simulink model "Prp_TrqDesCoord1"  (R2016b)
settings: configuration reference "CodeGenConfigSet" (kept outside this file)
settings Model: Creator=Wollf  LastModifiedBy=Wollf
settings ConfigSetRef: SourceLocation=Base Workspace

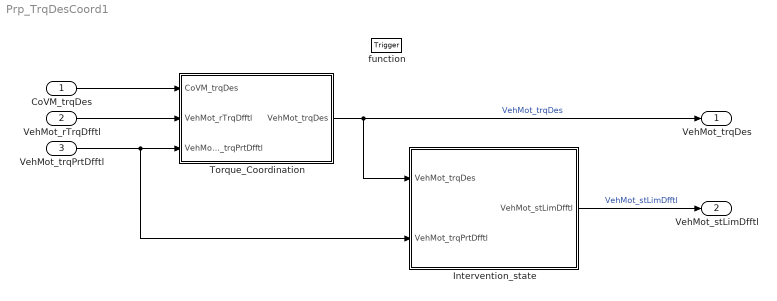
== system Prp_TrqDesCoord1 ==
  CoVM_trqDes : Inport  Tag=Nm  Description=Propulsion torque order after ESP-torque intervention coordination (wheel torque)  OutMin=-3000  OutMax=3000  OutDataTypeStr=Trq_Nm
  VehMot_rTrqDfftl : Inport  Description=Torque ratio of differential  Port=2  OutMin=-300  OutMax=300  OutDataTypeStr=TransRatio
  VehMot_trqPrtDfftl : Inport  Tag=Nm  Description=Differential protection torque  Port=3  OutMin=-3000  OutMax=3000  OutDataTypeStr=Trq_Nm
  function : TriggerPort  TriggerType=function-call  VariantControl=Variant
  Intervention_state : Subsystem
  Torque_Coordination : Subsystem
  VehMot_trqDes : Outport  Tag=Nm  Description=Desired torque for propulsion (transmission output torque)  OutMin=-3000  OutMax=3000  OutDataTypeStr=Trq_Nm
  VehMot_stLimDfftl : Outport  Description=Status torque intervention differential protection  Port=2  OutMin=0  OutMax=255  OutDataTypeStr=State_uint8
  wires:
  Intervention_state/1(VehMot_stLimDfftl) -> VehMot_stLimDfftl/1  "VehMot_stLimDfftl"
  CoVM_trqDes/1 -> Torque_Coordination/1(CoVM_trqDes)
  VehMot_rTrqDfftl/1 -> Torque_Coordination/2(VehMot_rTrqDfftl)
  VehMot_trqPrtDfftl/1 -> Intervention_state/2(VehMot_trqPrtDfftl), Torque_Coordination/3(VehMot_trqPrtDfftl)
  Torque_Coordination/1(VehMot_trqDes) -> VehMot_trqDes/1, Intervention_state/1(VehMot_trqDes)  "VehMot_trqDes"

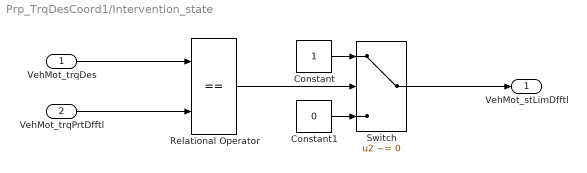
== system Prp_TrqDesCoord1/Intervention_state ==
  VehMot_trqDes : Inport
  VehMot_trqPrtDfftl : Inport  Port=2
  Constant : Constant  OutDataTypeStr=Inherit: Inherit via back propagation
  Constant1 : Constant  Value=0  OutDataTypeStr=Inherit: Inherit via back propagation
  Relational Operator : RelationalOperator  Operator===  OutDataTypeStr=boolean  RndMeth=Simplest  InputSameDT=on
  Switch : Switch  Criteria=u2 ~= 0  InputSameDT=on
  VehMot_stLimDfftl : Outport
  wires:
  Switch/1 -> VehMot_stLimDfftl/1
  Constant1/1 -> Switch/3
  Constant/1 -> Switch/1
  Relational Operator/1 -> Switch/2
  VehMot_trqPrtDfftl/1 -> Relational Operator/2
  VehMot_trqDes/1 -> Relational Operator/1

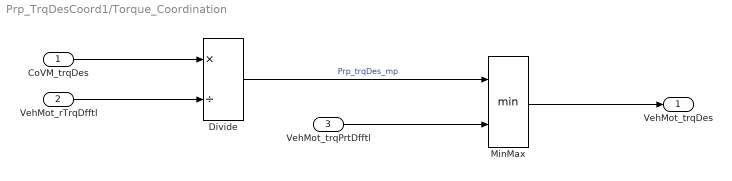
== system Prp_TrqDesCoord1/Torque_Coordination ==
  CoVM_trqDes : Inport  Tag=Nm  Description=Propulsion torque order after ESP-torque intervention coordination (wheel torque)  OutMin=-3000  OutMax=3000  OutDataTypeStr=Trq_Nm
  VehMot_rTrqDfftl : Inport  Tag=-  Description=Torque ratio of differential  Port=2  OutMin=-300  OutMax=300  OutDataTypeStr=TransRatio
  VehMot_trqPrtDfftl : Inport  Tag=Nm  Description=Differential protection torque  Port=3  OutMin=-3000  OutMax=3000  OutDataTypeStr=Trq_Nm
  Divide : Product  Inputs=*/  OutDataTypeStr=Trq_Nm
  MinMax : MinMax  Inputs=2  InputSameDT=on
  VehMot_trqDes : Outport
  wires:
  VehMot_trqPrtDfftl/1 -> MinMax/2
  CoVM_trqDes/1 -> Divide/1
  Divide/1 -> MinMax/1  "Prp_trqDes_mp"
  VehMot_rTrqDfftl/1 -> Divide/2
  MinMax/1 -> VehMot_trqDes/1
